simulink model "FF_Disturbance_simulink"  (R2018b)
settings: Solver=VariableStepAuto  StartTime=0.0  StopTime=12  RelTol=1e-3
undefined symbols (not defined in the file): alpha, CL, Cm, g, Iyy, m, V, varMass
libraries: vrlib x5, simulink_extras x2
settings Model: Creator=ferra  LastModifiedBy=ferra

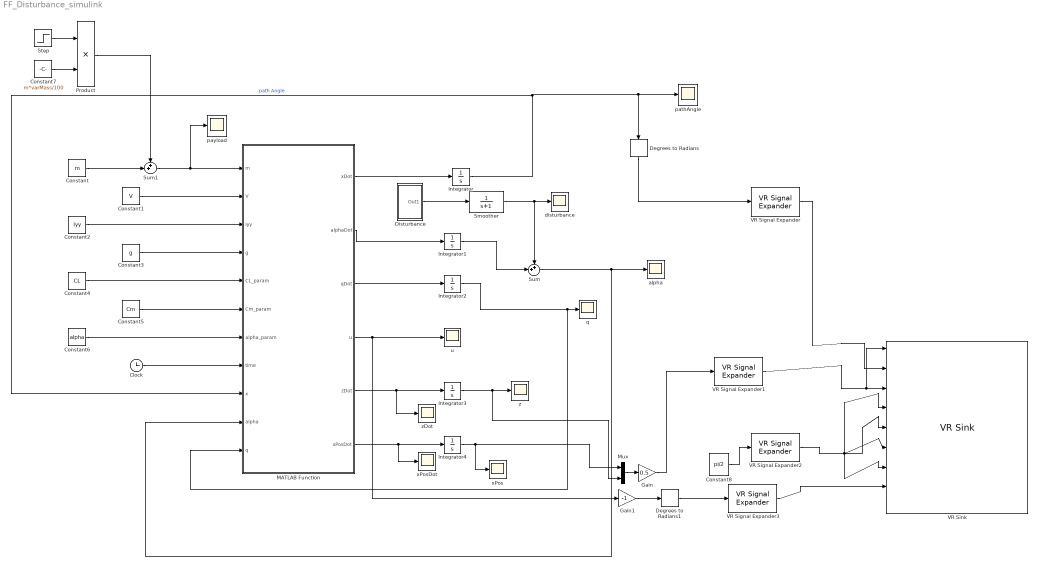
== system FF_Disturbance_simulink ==
  Clock : Clock
  Constant : Constant  Value=m
  Constant1 : Constant  Value=V
  Constant2 : Constant  Value=Iyy
  Constant3 : Constant  Value=g
  Constant4 : Constant  Value=CL
  Constant5 : Constant  Value=Cm
  Constant6 : Constant  Value=alpha
  Constant7 : Constant  Value=m*varMass/100
  Constant8 : Constant  Value=pi/2
  Degrees to Radians : simulink_extras/Transformations/Degrees to Radians
  Degrees to Radians1 : simulink_extras/Transformations/Degrees to Radians
  "Disturbance " : Subsystem
  Gain : Gain  Gain=0.5
  Gain1 : Gain  Gain=-1
  Integrator : Integrator
  Integrator1 : Integrator
  Integrator2 : Integrator
  Integrator3 : Integrator  InitialCondition=5
  Integrator4 : Integrator  InitialCondition=-70
  MATLAB Function : MATLAB Function  TreatAsAtomicUnit=on
  Mux : Mux  Inputs=2
  Product : Product
  "Smoother " : TransferFcn  Denominator=[1 1]
  Step : Step  Time=5  SampleTime=0
  Sum : Sum  Inputs=++|
  Sum1 : Sum  Inputs=++|
  VR Signal Expander : vrlib/VR Signal Expander  outwidth=4  outidx=[4]
      settings: SourceProductName=Simulink 3D Animation  SourceProductBaseCode=VR
  VR Signal Expander1 : vrlib/VR Signal Expander  outwidth=3  outidx=[1 2]
      settings: SourceProductName=Simulink 3D Animation  SourceProductBaseCode=VR
  VR Signal Expander2 : vrlib/VR Signal Expander  outwidth=4  outidx=[4]
      settings: SourceProductName=Simulink 3D Animation  SourceProductBaseCode=VR
  VR Signal Expander3 : vrlib/VR Signal Expander  outwidth=4  outidx=[4]
      settings: SourceProductName=Simulink 3D Animation  SourceProductBaseCode=VR
  VR Sink : vrlib/VR Sink  InstantiateOnLoad=on  SampleTime=0.05  ViewEnable=on  RemoteChange=off  RemoteView=off  FieldsWritten=FarAway_Front.position.3.1.1.double#Airplane.rotation.4.1.1.double#Airplane.translation.3.1.1.double#Rotor_1.rotation.4.1.1.double#Rotor_2.rotation.4.1.1.double#Rotor_3.rotation.4.1.1.double#Rotor_4.rotation.4.1.1.double#Flap_tail.rotation.4.1.1.double#Follow_Airplane.orientation.4.1.1.double  WorldFileName=C:\Users\ferra\Desktop\Projects\Matlab\Thesis\3D-simulation\3D_world.WRL  WorldDescription=Follow airplane  AutoView=off  VideoDimensions=[]  AllowVariableSize=off  FigureProperties="{'Position', 'Name', 'Viewpoint', 'CameraBound', 'CameraDirection', 'CameraPosition', 'CameraUpVector', 'ZoomFactor', 'Antialiasing', 'Headlight', 'Lighting', 'NavPanel', 'Sound', 'StatusBar', 'Stereo3D', 'Stereo3DCameraOffset', 'Stereo3DHIT', 'ToolBar', 'Textures', 'Transparency', 'Triad', 'Wireframe', 'NavZones', 'NavMode', 'NavSpeed', 'CaptureFileFormat', 'CaptureFileName', 'Record2DCompressMethod', 'Record2DCompressQuality', 'Record2D', 'Record2DFileName', 'Record2DFPS'; [1.0000000000000000e+00   7.6000000000000000e+01   1.9200000000000000e+03   9.5300000000000000e+02], 'Follow airplane', 'far away front POV', 'on', [-6.6932106743090844e-02  -3.9340503518798076e-01  -9.1692560841961179e-01], [6.4741097379861223e-01   3.1023324648929131e+00  -1.9803438957038846e+01], [9.1047643126099809e-03   9.1870732284332590e-01  -3.9483408948678772e-01], [1.0000000000000000e+00], 'on', 'on', 'on', 'halfbar', 'on', 'on', 'off', [1.0000000149011612e-01], [0.0000000000000000e+00], 'on', 'on', 'on', 'none', 'off', 'off', 'examine', 'normal', 'tif', '%f_anim_%n.tif', 'auto', [7.5000000000000000e+01], 'on', 'C:\\Users\\ferra\\Desktop\\Projects\\Matlab\\Thesis\\Recording_simulaiton\\FF_dist_pathAngle_mass.avi', [6.0000000000000000e+01]}"
      settings: SourceProductBaseCode=VR
  alpha : Scope
  disturbance : Scope
  pathAngle : Scope
  "payload " : Scope
  q : Scope
  u : Scope
  xPos : Scope
  xPosDot : Scope
  "z " : Scope
  zDot : Scope
  wires:
  Constant8/1 -> VR Signal Expander2/1
  MATLAB Function/1(xDot) -> Integrator/1
  Constant4/1 -> MATLAB Function/5(CL_param)
  Clock/1 -> MATLAB Function/8(time)
  Constant6/1 -> MATLAB Function/7(alpha_param)
  Integrator2/1 -> MATLAB Function/11(q), q/1
  Integrator/1 -> pathAngle/1, Degrees to Radians/1, MATLAB Function/9(x)  "path Angle"
  Integrator1/1 -> Sum/2
  "Disturbance "/1(Out1) -> "Smoother "/1
  "Smoother "/1 -> Sum/1, disturbance/1
  Gain1/1 -> Degrees to Radians1/1
  Constant3/1 -> MATLAB Function/4(g)
  MATLAB Function/4(u) -> Gain1/1, u/1
  Sum/1 -> MATLAB Function/10(alpha), alpha/1
  Constant7/1 -> Product/2
  MATLAB Function/3(qDot) -> Integrator2/1
  Constant2/1 -> MATLAB Function/3(Iyy)
  Gain/1 -> VR Signal Expander1/1
  Mux/1 -> Gain/1
  Degrees to Radians/1 -> VR Signal Expander/1
  Product/1 -> Sum1/1
  Integrator4/1 -> Mux/1, xPos/1
  Constant5/1 -> MATLAB Function/6(Cm_param)
  MATLAB Function/2(alphaDot) -> Integrator1/1
  Sum1/1 -> "payload "/1, MATLAB Function/1(m)
  MATLAB Function/6(xPosDot) -> xPosDot/1, Integrator4/1
  Constant1/1 -> MATLAB Function/2(V)
  Integrator3/1 -> Mux/2, "z "/1
  Step/1 -> Product/1
  Degrees to Radians1/1 -> VR Signal Expander3/1
  MATLAB Function/5(zDot) -> zDot/1, Integrator3/1
  Constant/1 -> Sum1/2
  VR Signal Expander/1 -> VR Sink/2
  VR Signal Expander1/1 -> VR Sink/1, VR Sink/3
  VR Signal Expander2/1 -> VR Sink/4, VR Sink/5, VR Sink/6, VR Sink/7
  VR Signal Expander3/1 -> VR Sink/8

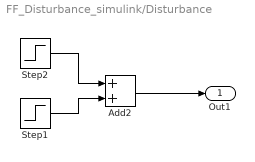
== system FF_Disturbance_simulink/Disturbance  ==
  Add2 : Sum
  Step1 : Step  Time=5  After=-20  SampleTime=0
  Step2 : Step  Time=3  After=20  SampleTime=0
  Out1 : Outport
  wires:
  Step2/1 -> Add2/1
  Step1/1 -> Add2/2
  Add2/1 -> Out1/1

== matlab function FF_Disturbance_simulink/MATLAB Function ==
  data: m input; xDot output; V input; Iyy input; g input; CL_param input; Cm_param input; alpha_param input; time input; alphaDot output; qDot output; x input; alpha input; q input; u output; zDot output; xPosDot output
function [xDot,alphaDot,qDot,u ,zDot , xPosDot ] = FF(m,V,Iyy,g,CL_param,Cm_param,...
                                    alpha_param, time,x,alpha,q)
Cm = mean(Cm_param);
T = 10;


k1 = 2;
k2 = 2;

if(alpha>71)
    alpha = 71;
elseif(alpha<-10)
    alpha = -10;
end



alphaRound = round(alpha*2)/2;

seqIndex = 1:1:length(alpha_param);
index = round(interp1(alpha_param,seqIndex,alphaRound));
CL = CL_param(index);

f = (-g/V) * cos((CL*x)/(m*V));
f1 = (g/V) * cos((CL*x)/(m*V)) - (CL*alpha)/(m*V);
f2 = 0;
g2 = Cm/Iyy;



df_dx =( (g*CL)/(m*V^2) ) * sin((CL*x)/(m*V));
df1_dx = ((-g*CL)/(m*V^2) ) *sin((CL*x)/(m*V));
df_ddx = ((g*CL^2)/(m*V^3)) * cos((CL * x)/(m*V));

%Definition of the xDes
amp = 1;
freq = 2*pi/10;
% xDes = amp * sin(freq*time);

xDes = 5;

e = x-xDes;

% xDesDot = amp *cos(freq*time);
xDesDot = 0;
alphaDes = -f - k1*e + xDesDot; %Virtual : stabilaize the dynamics of x 
alphaDesDot = (-df_dx -k1)*(f+alpha);


e1 = alpha - alphaDes;
qDes = -f1 -x+xDes - k1*e1 + alphaDesDot; %Virtual: stabilize the dynamics of alpha

e2 = q - qDes;

e1Dot = -e - k1*e1 +e2;





d_alphaDesDot_dx = -df_ddx *f - (df_dx)^2 -df_ddx * alpha - k1*df_dx;
par_qDes_x = -df1_dx - 1 + d_alphaDesDot_dx;
par_qDes_e1 = -k1;
qDesDot = par_qDes_x * (f+alpha) + par_qDes_e1 * (e1Dot);
u = (-f2 + qDesDot - e1 - k2*e2)/(g2);

xDot = f + alpha;
alphaDot = f1 + q;
qDot = f2 + g2 *u;
zDot  = V * sin(deg2rad(x));
xPosDot = V * cos(deg2rad(x));

end
